simulink model "simulacao"  (R2016a)
settings: Solver=ode45  StartTime=0.0  StopTime=800  RelTol=1e-3
undefined symbols (not defined in the file or in its folder): magnitude
libraries: simulink x12
settings Model: Creator=Paulo  LastModifiedBy=Nielsen
settings DataIOCC: LimitDataPoints=on  SaveFormat=Array
settings DebuggingCC: UnderspecifiedInitializationDetection=Classic  MergeDetectMultiDrivingBlocksExec=none  SolverPrmCheckMsg=warning  StateNameClashWarn=warning
settings HardwareCC: ProdBitPerPointer=32  ProdLargestAtomicFloat=None  ProdIntDivRoundTo=Undefined  ProdEndianess=Unspecified  ProdWordSize=32  ProdHWDeviceType=32-bit Generic
settings ModelReferenceCC: PropagateSignalLabelsOutOfModel=off
settings ConfigComp: CovModelRefEnable=Off

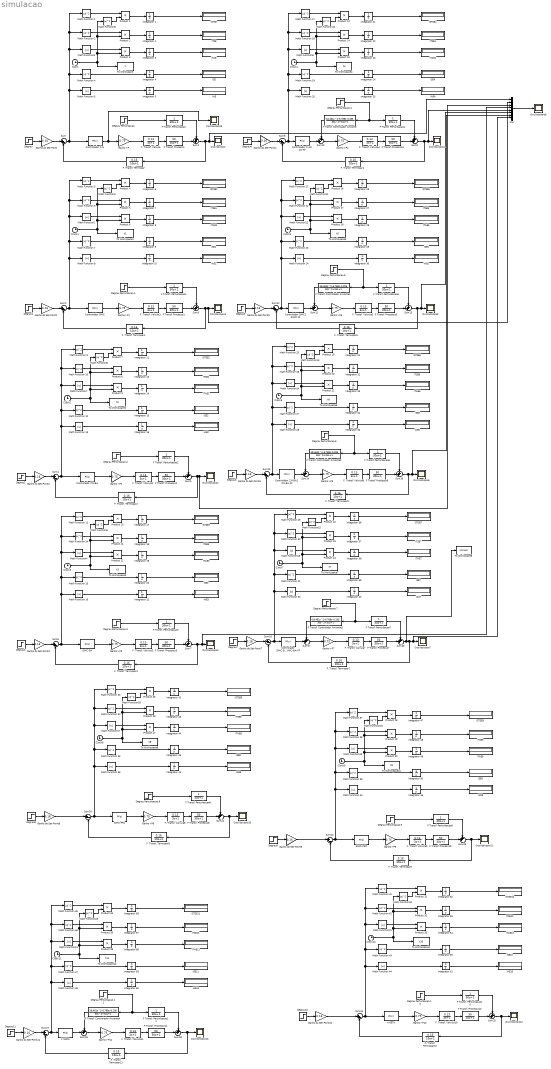
== system simulacao ==
  Clock{,1..11} (12 alike) : Clock
  Controlador SIMC : simulink/Continuous/PID Controller  Controller=PI  TimeDomain=Continuous-time  SampleTime=-1  IntegratorMethod=Forward Euler  FilterMethod=Forward Euler  Form=Parallel  UseFilter=on  ControllerParametersSource=internal  P=2.6618  I=0.0919  D=0  N=100  InitialConditionSource=internal  InitialConditionForIntegrator=0  InitialConditionForFilter=0  ExternalReset=none  LimitOutput=off  UpperSaturationLimit=10  LowerSaturationLimit=-10  LinearizeAsGain=on  AntiWindupMode=back-calculation  Kb=1  TrackingMode=off  Kt=1  PParamMin=[]  PParamMax=[]  IParamMin=[]  IParamMax=[]  DParamMin=[]  DParamMax=[]  NParamMin=[]  NParamMax=[]  KbParamMin=[]  KbParamMax=[]  KtParamMin=[]  KtParamMax=[]  POutMin=[]  POutMax=[]  IOutMin=[]  IOutMax=[]  DOutMin=[]  DOutMax=[]  NOutMin=[]  NOutMax=[]  KbOutMin=[]  KbOutMax=[]  KtOutMin=[]  KtOutMax=[]  IntegratorOutMin=[]  IntegratorOutMax=[]  FilterOutMin=[]  FilterOutMax=[]  SumOutMin=[]  SumOutMax=[]  SumI1OutMin=[]  SumI1OutMax=[]  SumI2OutMin=[]  SumI2OutMax=[]  SumI3OutMin=[]  SumI3OutMax=[]  SumDOutMin=[]  SumDOutMax=[]  SaturationOutMin=[]  SaturationOutMax=[]  IntegratorContinuousStateAttributes=''  IntegratorStateMustResolveToSignalObject=off  IntegratorRTWStateStorageClass=Auto  FilterContinuousStateAttributes=''  FilterStateMustResolveToSignalObject=off  FilterRTWStateStorageClass=Auto  DifferentiatorICPrevScaledInput=0  DifferentiatorOutMin=[]  DifferentiatorOutMax=[]
  Controlador SIMC-BA2 SIMIC-BA-FF : simulink/Continuous/PID Controller  Controller=PI  TimeDomain=Continuous-time  SampleTime=-1  IntegratorMethod=Forward Euler  FilterMethod=Forward Euler  Form=Parallel  UseFilter=on  ControllerParametersSource=internal  P=2.0483  I=0.054208  D=0  N=100  InitialConditionSource=internal  InitialConditionForIntegrator=0  InitialConditionForFilter=0  ExternalReset=none  LimitOutput=off  UpperSaturationLimit=10  LowerSaturationLimit=-10  LinearizeAsGain=on  AntiWindupMode=back-calculation  Kb=1  TrackingMode=off  Kt=1  PParamMin=[]  PParamMax=[]  IParamMin=[]  IParamMax=[]  DParamMin=[]  DParamMax=[]  NParamMin=[]  NParamMax=[]  KbParamMin=[]  KbParamMax=[]  KtParamMin=[]  KtParamMax=[]  POutMin=[]  POutMax=[]  IOutMin=[]  IOutMax=[]  DOutMin=[]  DOutMax=[]  NOutMin=[]  NOutMax=[]  KbOutMin=[]  KbOutMax=[]  KtOutMin=[]  KtOutMax=[]  IntegratorOutMin=[]  IntegratorOutMax=[]  FilterOutMin=[]  FilterOutMax=[]  SumOutMin=[]  SumOutMax=[]  SumI1OutMin=[]  SumI1OutMax=[]  SumI2OutMin=[]  SumI2OutMax=[]  SumI3OutMin=[]  SumI3OutMax=[]  SumDOutMin=[]  SumDOutMax=[]  SaturationOutMin=[]  SaturationOutMax=[]  IntegratorContinuousStateAttributes=''  IntegratorStateMustResolveToSignalObject=off  IntegratorRTWStateStorageClass=Auto  FilterContinuousStateAttributes=''  FilterStateMustResolveToSignalObject=off  FilterRTWStateStorageClass=Auto  DifferentiatorICPrevScaledInput=0  DifferentiatorOutMin=[]  DifferentiatorOutMax=[]
  "Controlador SIMC2 SIMIC FF " : simulink/Continuous/PID Controller  Controller=PI  TimeDomain=Continuous-time  SampleTime=-1  IntegratorMethod=Forward Euler  FilterMethod=Forward Euler  Form=Parallel  UseFilter=on  ControllerParametersSource=internal  P=2.6618  I=0.0919  D=0  N=100  InitialConditionSource=internal  InitialConditionForIntegrator=0  InitialConditionForFilter=0  ExternalReset=none  LimitOutput=off  UpperSaturationLimit=10  LowerSaturationLimit=-10  LinearizeAsGain=on  AntiWindupMode=back-calculation  Kb=1  TrackingMode=off  Kt=1  PParamMin=[]  PParamMax=[]  IParamMin=[]  IParamMax=[]  DParamMin=[]  DParamMax=[]  NParamMin=[]  NParamMax=[]  KbParamMin=[]  KbParamMax=[]  KtParamMin=[]  KtParamMax=[]  POutMin=[]  POutMax=[]  IOutMin=[]  IOutMax=[]  DOutMin=[]  DOutMax=[]  NOutMin=[]  NOutMax=[]  KbOutMin=[]  KbOutMax=[]  KtOutMin=[]  KtOutMax=[]  IntegratorOutMin=[]  IntegratorOutMax=[]  FilterOutMin=[]  FilterOutMax=[]  SumOutMin=[]  SumOutMax=[]  SumI1OutMin=[]  SumI1OutMax=[]  SumI2OutMin=[]  SumI2OutMax=[]  SumI3OutMin=[]  SumI3OutMax=[]  SumDOutMin=[]  SumDOutMax=[]  SaturationOutMin=[]  SaturationOutMax=[]  IntegratorContinuousStateAttributes=''  IntegratorStateMustResolveToSignalObject=off  IntegratorRTWStateStorageClass=Auto  FilterContinuousStateAttributes=''  FilterStateMustResolveToSignalObject=off  FilterRTWStateStorageClass=Auto  DifferentiatorICPrevScaledInput=0  DifferentiatorOutMin=[]  DifferentiatorOutMax=[]
  Controlador Z-N : simulink/Continuous/PID Controller  Controller=PI  TimeDomain=Continuous-time  SampleTime=-1  IntegratorMethod=Forward Euler  FilterMethod=Forward Euler  Form=Parallel  UseFilter=on  ControllerParametersSource=internal  P=10.71  I=0.437  D=0  N=100  InitialConditionSource=internal  InitialConditionForIntegrator=0  InitialConditionForFilter=0  ExternalReset=none  LimitOutput=off  UpperSaturationLimit=10  LowerSaturationLimit=-10  LinearizeAsGain=on  AntiWindupMode=back-calculation  Kb=1  TrackingMode=off  Kt=1  PParamMin=[]  PParamMax=[]  IParamMin=[]  IParamMax=[]  DParamMin=[]  DParamMax=[]  NParamMin=[]  NParamMax=[]  KbParamMin=[]  KbParamMax=[]  KtParamMin=[]  KtParamMax=[]  POutMin=[]  POutMax=[]  IOutMin=[]  IOutMax=[]  DOutMin=[]  DOutMax=[]  NOutMin=[]  NOutMax=[]  KbOutMin=[]  KbOutMax=[]  KtOutMin=[]  KtOutMax=[]  IntegratorOutMin=[]  IntegratorOutMax=[]  FilterOutMin=[]  FilterOutMax=[]  SumOutMin=[]  SumOutMax=[]  SumI1OutMin=[]  SumI1OutMax=[]  SumI2OutMin=[]  SumI2OutMax=[]  SumI3OutMin=[]  SumI3OutMax=[]  SumDOutMin=[]  SumDOutMax=[]  SaturationOutMin=[]  SaturationOutMax=[]  IntegratorContinuousStateAttributes=''  IntegratorStateMustResolveToSignalObject=off  IntegratorRTWStateStorageClass=Auto  FilterContinuousStateAttributes=''  FilterStateMustResolveToSignalObject=off  FilterRTWStateStorageClass=Auto  DifferentiatorICPrevScaledInput=0  DifferentiatorOutMin=[]  DifferentiatorOutMax=[]
  Controlador Z-N2 ZN-FF : simulink/Continuous/PID Controller  Controller=PI  TimeDomain=Continuous-time  SampleTime=-1  IntegratorMethod=Forward Euler  FilterMethod=Forward Euler  Form=Parallel  UseFilter=on  ControllerParametersSource=internal  P=10.71  I=0.437  D=0  N=100  InitialConditionSource=internal  InitialConditionForIntegrator=0  InitialConditionForFilter=0  ExternalReset=none  LimitOutput=off  UpperSaturationLimit=10  LowerSaturationLimit=-10  LinearizeAsGain=on  AntiWindupMode=back-calculation  Kb=1  TrackingMode=off  Kt=1  PParamMin=[]  PParamMax=[]  IParamMin=[]  IParamMax=[]  DParamMin=[]  DParamMax=[]  NParamMin=[]  NParamMax=[]  KbParamMin=[]  KbParamMax=[]  KtParamMin=[]  KtParamMax=[]  POutMin=[]  POutMax=[]  IOutMin=[]  IOutMax=[]  DOutMin=[]  DOutMax=[]  NOutMin=[]  NOutMax=[]  KbOutMin=[]  KbOutMax=[]  KtOutMin=[]  KtOutMax=[]  IntegratorOutMin=[]  IntegratorOutMax=[]  FilterOutMin=[]  FilterOutMax=[]  SumOutMin=[]  SumOutMax=[]  SumI1OutMin=[]  SumI1OutMax=[]  SumI2OutMin=[]  SumI2OutMax=[]  SumI3OutMin=[]  SumI3OutMax=[]  SumDOutMin=[]  SumDOutMax=[]  SaturationOutMin=[]  SaturationOutMax=[]  IntegratorContinuousStateAttributes=''  IntegratorStateMustResolveToSignalObject=off  IntegratorRTWStateStorageClass=Auto  FilterContinuousStateAttributes=''  FilterStateMustResolveToSignalObject=off  FilterRTWStateStorageClass=Auto  DifferentiatorICPrevScaledInput=0  DifferentiatorOutMin=[]  DifferentiatorOutMax=[]
  Controlador ZN-BA : simulink/Continuous/PID Controller  Controller=PI  TimeDomain=Continuous-time  SampleTime=-1  IntegratorMethod=Forward Euler  FilterMethod=Forward Euler  Form=Parallel  UseFilter=on  ControllerParametersSource=internal  P=5.355  I=0.2185  D=0  N=100  InitialConditionSource=internal  InitialConditionForIntegrator=0  InitialConditionForFilter=0  ExternalReset=none  LimitOutput=off  UpperSaturationLimit=10  LowerSaturationLimit=-10  LinearizeAsGain=on  AntiWindupMode=back-calculation  Kb=1  TrackingMode=off  Kt=1  PParamMin=[]  PParamMax=[]  IParamMin=[]  IParamMax=[]  DParamMin=[]  DParamMax=[]  NParamMin=[]  NParamMax=[]  KbParamMin=[]  KbParamMax=[]  KtParamMin=[]  KtParamMax=[]  POutMin=[]  POutMax=[]  IOutMin=[]  IOutMax=[]  DOutMin=[]  DOutMax=[]  NOutMin=[]  NOutMax=[]  KbOutMin=[]  KbOutMax=[]  KtOutMin=[]  KtOutMax=[]  IntegratorOutMin=[]  IntegratorOutMax=[]  FilterOutMin=[]  FilterOutMax=[]  SumOutMin=[]  SumOutMax=[]  SumI1OutMin=[]  SumI1OutMax=[]  SumI2OutMin=[]  SumI2OutMax=[]  SumI3OutMin=[]  SumI3OutMax=[]  SumDOutMin=[]  SumDOutMax=[]  SaturationOutMin=[]  SaturationOutMax=[]  IntegratorContinuousStateAttributes=''  IntegratorStateMustResolveToSignalObject=off  IntegratorRTWStateStorageClass=Auto  FilterContinuousStateAttributes=''  FilterStateMustResolveToSignalObject=off  FilterRTWStateStorageClass=Auto  DifferentiatorICPrevScaledInput=0  DifferentiatorOutMin=[]  DifferentiatorOutMax=[]
  Controlador ZN-BA2 ZN-BA-FF : simulink/Continuous/PID Controller  Controller=PI  TimeDomain=Continuous-time  SampleTime=-1  IntegratorMethod=Forward Euler  FilterMethod=Forward Euler  Form=Parallel  UseFilter=on  ControllerParametersSource=internal  P=5.355  I=0.2185  D=0  N=100  InitialConditionSource=internal  InitialConditionForIntegrator=0  InitialConditionForFilter=0  ExternalReset=none  LimitOutput=off  UpperSaturationLimit=10  LowerSaturationLimit=-10  LinearizeAsGain=on  AntiWindupMode=back-calculation  Kb=1  TrackingMode=off  Kt=1  PParamMin=[]  PParamMax=[]  IParamMin=[]  IParamMax=[]  DParamMin=[]  DParamMax=[]  NParamMin=[]  NParamMax=[]  KbParamMin=[]  KbParamMax=[]  KtParamMin=[]  KtParamMax=[]  POutMin=[]  POutMax=[]  IOutMin=[]  IOutMax=[]  DOutMin=[]  DOutMax=[]  NOutMin=[]  NOutMax=[]  KbOutMin=[]  KbOutMax=[]  KtOutMin=[]  KtOutMax=[]  IntegratorOutMin=[]  IntegratorOutMax=[]  FilterOutMin=[]  FilterOutMax=[]  SumOutMin=[]  SumOutMax=[]  SumI1OutMin=[]  SumI1OutMax=[]  SumI2OutMin=[]  SumI2OutMax=[]  SumI3OutMin=[]  SumI3OutMax=[]  SumDOutMin=[]  SumDOutMax=[]  SaturationOutMin=[]  SaturationOutMax=[]  IntegratorContinuousStateAttributes=''  IntegratorStateMustResolveToSignalObject=off  IntegratorRTWStateStorageClass=Auto  FilterContinuousStateAttributes=''  FilterStateMustResolveToSignalObject=off  FilterRTWStateStorageClass=Auto  DifferentiatorICPrevScaledInput=0  DifferentiatorOutMin=[]  DifferentiatorOutMax=[]
  Degrau{,1..11} (12 alike) : Step  Time=0  SampleTime=0
  Degrau Perturbacao.{,1..11} (12 alike) : Step  Time=0  SampleTime=0
  F Transf. Controlador Anvante{,1..4} (5 alike) : TransferFcn  Numerator=[-18.461 -6.769 -0.205]  Denominator=[30 31 1]
  F Transf. Perturbacao{,1..11} (12 alike) : TransferFcn  Denominator=[30 1]
  F Transf. Processo{,1..11} (12 alike) : TransferFcn  Numerator=[50]  Denominator=[30 1]
  F. Transf. Termopar{,1..11} (12 alike) : TransferFcn  Numerator=[0.16]  Denominator=[10 1]
  F. Transf. Válvula{,1..11} (12 alike) : TransferFcn  Numerator=[0.13]  Denominator=[3 1]
  Ganho I-P{,1..11} (12 alike) : Gain  Gain=0.75
  Ganho do Set-Point{,1..11} (12 alike) : Gain  Gain=0.16
  IAE{,1..11} (12 alike) : Display
  ISE{,1..11} (12 alike) : Display
  ISTSE{,1..11} (12 alike) : Display
  ITAE{,1..11} (12 alike) : Display
  ITSE{,1..11} (12 alike) : Display
  Integrator {1..60} (60 alike) : Integrator
  Math Function {1..4,6..7,9..12,14..15,17..19,21..23,25..27,29..31,33..35,37..39,41..43,45..47} (36 alike) : Math  Operator=magnitude^2  SaturateOnIntegerOverflow=on
  Math Function {5,8,13,16,20,24,28,32,36,40,44,48} (12 alike) : Abs
  Math Function{1,3..4,7,9,12,14,16..17,19,21,24} (12 alike) : Abs
  Math Function{2,5..6,8,10..11,13,15,18,20,22..23} (12 alike) : Math  Operator=magnitude^2  SaturateOnIntegerOverflow=on
  Mux : Mux  Inputs=8
  Osciloscópio{,1..13} (14 alike) : Scope
  Product {1..36} (36 alike) : Product
  SIMC-BA : simulink/Continuous/PID Controller  Controller=PI  TimeDomain=Continuous-time  SampleTime=-1  IntegratorMethod=Forward Euler  FilterMethod=Forward Euler  Form=Parallel  UseFilter=on  ControllerParametersSource=internal  P=2.0483  I=0.054208  D=0  N=100  InitialConditionSource=internal  InitialConditionForIntegrator=0  InitialConditionForFilter=0  ExternalReset=none  LimitOutput=off  UpperSaturationLimit=10  LowerSaturationLimit=-10  LinearizeAsGain=on  AntiWindupMode=back-calculation  Kb=1  TrackingMode=off  Kt=1  PParamMin=[]  PParamMax=[]  IParamMin=[]  IParamMax=[]  DParamMin=[]  DParamMax=[]  NParamMin=[]  NParamMax=[]  KbParamMin=[]  KbParamMax=[]  KtParamMin=[]  KtParamMax=[]  POutMin=[]  POutMax=[]  IOutMin=[]  IOutMax=[]  DOutMin=[]  DOutMax=[]  NOutMin=[]  NOutMax=[]  KbOutMin=[]  KbOutMax=[]  KtOutMin=[]  KtOutMax=[]  IntegratorOutMin=[]  IntegratorOutMax=[]  FilterOutMin=[]  FilterOutMax=[]  SumOutMin=[]  SumOutMax=[]  SumI1OutMin=[]  SumI1OutMax=[]  SumI2OutMin=[]  SumI2OutMax=[]  SumI3OutMin=[]  SumI3OutMax=[]  SumDOutMin=[]  SumDOutMax=[]  SaturationOutMin=[]  SaturationOutMax=[]  IntegratorContinuousStateAttributes=''  IntegratorStateMustResolveToSignalObject=off  IntegratorRTWStateStorageClass=Auto  FilterContinuousStateAttributes=''  FilterStateMustResolveToSignalObject=off  FilterRTWStateStorageClass=Auto  DifferentiatorICPrevScaledInput=0  DifferentiatorOutMin=[]  DifferentiatorOutMax=[]
  SIMC-FPA : simulink/Continuous/PID Controller  Controller=PI  TimeDomain=Continuous-time  SampleTime=-1  IntegratorMethod=Forward Euler  FilterMethod=Forward Euler  Form=Parallel  UseFilter=on  ControllerParametersSource=internal  P=5.7554  I=0.2185  D=0  N=100  InitialConditionSource=internal  InitialConditionForIntegrator=0  InitialConditionForFilter=0  ExternalReset=none  LimitOutput=off  UpperSaturationLimit=10  LowerSaturationLimit=-10  LinearizeAsGain=on  AntiWindupMode=back-calculation  Kb=1  TrackingMode=off  Kt=1  PParamMin=[]  PParamMax=[]  IParamMin=[]  IParamMax=[]  DParamMin=[]  DParamMax=[]  NParamMin=[]  NParamMax=[]  KbParamMin=[]  KbParamMax=[]  KtParamMin=[]  KtParamMax=[]  POutMin=[]  POutMax=[]  IOutMin=[]  IOutMax=[]  DOutMin=[]  DOutMax=[]  NOutMin=[]  NOutMax=[]  KbOutMin=[]  KbOutMax=[]  KtOutMin=[]  KtOutMax=[]  IntegratorOutMin=[]  IntegratorOutMax=[]  FilterOutMin=[]  FilterOutMax=[]  SumOutMin=[]  SumOutMax=[]  SumI1OutMin=[]  SumI1OutMax=[]  SumI2OutMin=[]  SumI2OutMax=[]  SumI3OutMin=[]  SumI3OutMax=[]  SumDOutMin=[]  SumDOutMax=[]  SaturationOutMin=[]  SaturationOutMax=[]  IntegratorContinuousStateAttributes=''  IntegratorStateMustResolveToSignalObject=off  IntegratorRTWStateStorageClass=Auto  FilterContinuousStateAttributes=''  FilterStateMustResolveToSignalObject=off  FilterRTWStateStorageClass=Auto  DifferentiatorICPrevScaledInput=0  DifferentiatorOutMin=[]  DifferentiatorOutMax=[]
  SIMC-PSO : simulink/Continuous/PID Controller  Controller=PI  TimeDomain=Continuous-time  SampleTime=-1  IntegratorMethod=Forward Euler  FilterMethod=Forward Euler  Form=Parallel  UseFilter=on  ControllerParametersSource=internal  P=1.8638  I=0.0505  D=0  N=100  InitialConditionSource=internal  InitialConditionForIntegrator=0  InitialConditionForFilter=0  ExternalReset=none  LimitOutput=off  UpperSaturationLimit=10  LowerSaturationLimit=-10  LinearizeAsGain=on  AntiWindupMode=back-calculation  Kb=1  TrackingMode=off  Kt=1  PParamMin=[]  PParamMax=[]  IParamMin=[]  IParamMax=[]  DParamMin=[]  DParamMax=[]  NParamMin=[]  NParamMax=[]  KbParamMin=[]  KbParamMax=[]  KtParamMin=[]  KtParamMax=[]  POutMin=[]  POutMax=[]  IOutMin=[]  IOutMax=[]  DOutMin=[]  DOutMax=[]  NOutMin=[]  NOutMax=[]  KbOutMin=[]  KbOutMax=[]  KtOutMin=[]  KtOutMax=[]  IntegratorOutMin=[]  IntegratorOutMax=[]  FilterOutMin=[]  FilterOutMax=[]  SumOutMin=[]  SumOutMax=[]  SumI1OutMin=[]  SumI1OutMax=[]  SumI2OutMin=[]  SumI2OutMax=[]  SumI3OutMin=[]  SumI3OutMax=[]  SumDOutMin=[]  SumDOutMax=[]  SaturationOutMin=[]  SaturationOutMax=[]  IntegratorContinuousStateAttributes=''  IntegratorStateMustResolveToSignalObject=off  IntegratorRTWStateStorageClass=Auto  FilterContinuousStateAttributes=''  FilterStateMustResolveToSignalObject=off  FilterRTWStateStorageClass=Auto  DifferentiatorICPrevScaledInput=0  DifferentiatorOutMin=[]  DifferentiatorOutMax=[]
  Sum{,2,4,6,8,12,15,18,20,22,24,27} (12 alike) : Sum  Inputs=|+-
  Sum{1,3,5,7,9..11,13..14,16..17,19,21,23,25..26,28} (17 alike) : Sum  Inputs=++|
  To Workspace : ToWorkspace  VariableName=t  SampleTime=-1
  To Workspace1 : ToWorkspace  VariableName=t1  SampleTime=-1
  To Workspace10 : ToWorkspace  VariableName=t9  SampleTime=-1
  To Workspace11 : ToWorkspace  VariableName=t10  SampleTime=-1
  To Workspace12 : ToWorkspace  VariableName=t11  SampleTime=-1
  To Workspace2 : ToWorkspace  VariableName=t2  SampleTime=-1
  To Workspace3 : ToWorkspace  VariableName=t3  SampleTime=-1
  To Workspace4 : ToWorkspace  VariableName=t4  SampleTime=-1
  To Workspace5 : ToWorkspace  VariableName=t5  SampleTime=-1
  To Workspace6 : ToWorkspace  VariableName=t6  SampleTime=-1
  To Workspace7 : ToWorkspace  VariableName=t7  SampleTime=-1
  To Workspace8 : ToWorkspace  VariableName=simout  SampleTime=-1
  To Workspace9 : ToWorkspace  VariableName=t8  SampleTime=-1
  X META : simulink/Continuous/PID Controller  Controller=PI  TimeDomain=Continuous-time  SampleTime=-1  IntegratorMethod=Forward Euler  FilterMethod=Forward Euler  Form=Parallel  UseFilter=on  ControllerParametersSource=internal  P=10.71  I=0.437  D=0  N=100  InitialConditionSource=internal  InitialConditionForIntegrator=0  InitialConditionForFilter=0  ExternalReset=none  LimitOutput=off  UpperSaturationLimit=10  LowerSaturationLimit=-10  LinearizeAsGain=on  AntiWindupMode=back-calculation  Kb=1  TrackingMode=off  Kt=1  PParamMin=[]  PParamMax=[]  IParamMin=[]  IParamMax=[]  DParamMin=[]  DParamMax=[]  NParamMin=[]  NParamMax=[]  KbParamMin=[]  KbParamMax=[]  KtParamMin=[]  KtParamMax=[]  POutMin=[]  POutMax=[]  IOutMin=[]  IOutMax=[]  DOutMin=[]  DOutMax=[]  NOutMin=[]  NOutMax=[]  KbOutMin=[]  KbOutMax=[]  KtOutMin=[]  KtOutMax=[]  IntegratorOutMin=[]  IntegratorOutMax=[]  FilterOutMin=[]  FilterOutMax=[]  SumOutMin=[]  SumOutMax=[]  SumI1OutMin=[]  SumI1OutMax=[]  SumI2OutMin=[]  SumI2OutMax=[]  SumI3OutMin=[]  SumI3OutMax=[]  SumDOutMin=[]  SumDOutMax=[]  SaturationOutMin=[]  SaturationOutMax=[]  IntegratorContinuousStateAttributes=''  IntegratorStateMustResolveToSignalObject=off  IntegratorRTWStateStorageClass=Auto  FilterContinuousStateAttributes=''  FilterStateMustResolveToSignalObject=off  FilterRTWStateStorageClass=Auto  DifferentiatorICPrevScaledInput=0  DifferentiatorOutMin=[]  DifferentiatorOutMax=[]
  XMETA : simulink/Continuous/PID Controller  Controller=PI  TimeDomain=Continuous-time  SampleTime=-1  IntegratorMethod=Forward Euler  FilterMethod=Forward Euler  Form=Parallel  UseFilter=on  ControllerParametersSource=internal  P=5.2114  I=0.1140  D=0  N=100  InitialConditionSource=internal  InitialConditionForIntegrator=0  InitialConditionForFilter=0  ExternalReset=none  LimitOutput=off  UpperSaturationLimit=10  LowerSaturationLimit=-10  LinearizeAsGain=on  AntiWindupMode=back-calculation  Kb=1  TrackingMode=off  Kt=1  PParamMin=[]  PParamMax=[]  IParamMin=[]  IParamMax=[]  DParamMin=[]  DParamMax=[]  NParamMin=[]  NParamMax=[]  KbParamMin=[]  KbParamMax=[]  KtParamMin=[]  KtParamMax=[]  POutMin=[]  POutMax=[]  IOutMin=[]  IOutMax=[]  DOutMin=[]  DOutMax=[]  NOutMin=[]  NOutMax=[]  KbOutMin=[]  KbOutMax=[]  KtOutMin=[]  KtOutMax=[]  IntegratorOutMin=[]  IntegratorOutMax=[]  FilterOutMin=[]  FilterOutMax=[]  SumOutMin=[]  SumOutMax=[]  SumI1OutMin=[]  SumI1OutMax=[]  SumI2OutMin=[]  SumI2OutMax=[]  SumI3OutMin=[]  SumI3OutMax=[]  SumDOutMin=[]  SumDOutMax=[]  SaturationOutMin=[]  SaturationOutMax=[]  IntegratorContinuousStateAttributes=''  IntegratorStateMustResolveToSignalObject=off  IntegratorRTWStateStorageClass=Auto  FilterContinuousStateAttributes=''  FilterStateMustResolveToSignalObject=off  FilterRTWStateStorageClass=Auto  DifferentiatorICPrevScaledInput=0  DifferentiatorOutMin=[]  DifferentiatorOutMax=[]
  wires:
  Degrau/1 -> Ganho do Set-Point/1
  Ganho do Set-Point/1 -> Sum/1
  Ganho I-P/1 -> F. Transf. Válvula/1
  F. Transf. Válvula/1 -> F Transf. Processo/1
  F. Transf. Termopar/1 -> Sum/2
  F Transf. Perturbacao/1 -> Sum1/1
  F Transf. Processo/1 -> Sum1/2
  Degrau Perturbacao./1 -> F Transf. Perturbacao/1
  Sum/1 -> Math Function 5/1, Math Function 4/1, Math Function3/1, Math Function 2/1, Math Function 1/1, Controlador Z-N/1
  Product 1/1 -> Integrator 1/1
  Product 2/1 -> Integrator 2/1
  Product 3/1 -> Integrator 3/1
  Math Function3/1 -> Product 3/1
  Math Function 1/1 -> Product 1/1
  Math Function 2/1 -> Product 2/1
  Integrator 1/1 -> ISTSE/1
  Integrator 2/1 -> ITSE/1
  Integrator 3/1 -> ITAE/1
  Math Function 4/1 -> Integrator 4/1
  Math Function 5/1 -> Integrator 5/1
  Clock/1 -> Product 3/2, Product 2/2, Math Function6/1, To Workspace/1
  Math Function6/1 -> Product 1/2
  Integrator 4/1 -> ISE/1
  Integrator 5/1 -> IAE/1
  Degrau1/1 -> Ganho do Set-Point1/1
  Ganho do Set-Point1/1 -> Sum2/1
  Ganho I-P1/1 -> F. Transf. Válvula1/1
  F. Transf. Válvula1/1 -> F Transf. Processo1/1
  F. Transf. Termopar1/1 -> Sum2/2
  F Transf. Perturbacao1/1 -> Sum3/1
  F Transf. Processo1/1 -> Sum3/2
  Degrau Perturbacao.1/1 -> F Transf. Perturbacao1/1
  Sum2/1 -> Math Function 8/1, Math Function 7/1, Math Function1/1, Math Function 6/1, Math Function 3/1, Controlador SIMC/1
  Product 4/1 -> Integrator 6/1
  Product 5/1 -> Integrator 7/1
  Product 6/1 -> Integrator 8/1
  Math Function1/1 -> Product 6/1
  Math Function 3/1 -> Product 4/1
  Math Function 6/1 -> Product 5/1
  Integrator 6/1 -> ISTSE1/1
  Integrator 7/1 -> ITSE1/1
  Integrator 8/1 -> ITAE1/1
  Math Function 7/1 -> Integrator 9/1
  Math Function 8/1 -> Integrator 10/1
  Clock1/1 -> Product 6/2, Product 5/2, Math Function2/1, To Workspace1/1
  Math Function2/1 -> Product 4/2
  Integrator 9/1 -> ISE1/1
  Integrator 10/1 -> IAE1/1
  Controlador SIMC/1 -> Ganho I-P1/1
  Degrau2/1 -> Ganho do Set-Point2/1
  Ganho do Set-Point2/1 -> Sum4/1
  Ganho I-P2/1 -> F. Transf. Válvula2/1
  F. Transf. Válvula2/1 -> F Transf. Processo2/1
  F. Transf. Termopar2/1 -> Sum4/2
  F Transf. Perturbacao2/1 -> Sum5/1
  F Transf. Processo2/1 -> Sum5/2
  Degrau Perturbacao.2/1 -> F Transf. Perturbacao2/1
  Sum4/1 -> Math Function 13/1, Math Function 12/1, Math Function7/1, Math Function 10/1, Math Function 9/1, Controlador ZN-BA/1
  Product 7/1 -> Integrator 11/1
  Product 8/1 -> Integrator 13/1
  Product 9/1 -> Integrator 14/1
  Math Function7/1 -> Product 9/1
  Math Function 9/1 -> Product 7/1
  Math Function 10/1 -> Product 8/1
  Integrator 11/1 -> ISTSE2/1
  Integrator 13/1 -> ITSE2/1
  Integrator 14/1 -> ITAE2/1
  Math Function 12/1 -> Integrator 15/1
  Math Function 13/1 -> Integrator 16/1
  Clock2/1 -> Product 9/2, Product 8/2, Math Function8/1, To Workspace2/1
  Math Function8/1 -> Product 7/2
  Integrator 15/1 -> ISE2/1
  Integrator 16/1 -> IAE2/1
  Controlador ZN-BA/1 -> Ganho I-P2/1
  Degrau3/1 -> Ganho do Set-Point3/1
  Ganho do Set-Point3/1 -> Sum6/1
  Ganho I-P3/1 -> F. Transf. Válvula3/1
  F. Transf. Válvula3/1 -> F Transf. Processo3/1
  F. Transf. Termopar3/1 -> Sum6/2
  F Transf. Processo3/1 -> Sum7/2
  Degrau Perturbacao.3/1 -> F Transf. Perturbacao3/1
  Sum6/1 -> Math Function 16/1, Math Function 15/1, Math Function4/1, Math Function 14/1, Math Function 11/1, SIMC-BA/1
  Product 10/1 -> Integrator 17/1
  Product 11/1 -> Integrator 18/1
  Product 12/1 -> Integrator 19/1
  Math Function4/1 -> Product 12/1
  Math Function 11/1 -> Product 10/1
  Math Function 14/1 -> Product 11/1
  Integrator 17/1 -> ISTSE3/1
  Integrator 18/1 -> ITSE3/1
  Integrator 19/1 -> ITAE3/1
  Math Function 15/1 -> Integrator 20/1
  Math Function 16/1 -> Integrator 12/1
  Clock3/1 -> Product 12/2, Product 11/2, Math Function5/1, To Workspace3/1
  Math Function5/1 -> Product 10/2
  Integrator 20/1 -> ISE3/1
  Integrator 12/1 -> IAE3/1
  SIMC-BA/1 -> Ganho I-P3/1
  Degrau4/1 -> Ganho do Set-Point4/1
  Ganho do Set-Point4/1 -> Sum8/1
  Ganho I-P4/1 -> F. Transf. Válvula4/1
  F. Transf. Válvula4/1 -> F Transf. Processo4/1
  F. Transf. Termopar4/1 -> Sum8/2
  F Transf. Perturbacao4/1 -> Sum9/1
  Sum10/1 -> Ganho I-P4/1
  Controlador Z-N2 ZN-FF/1 -> Sum10/2
  F Transf. Controlador Anvante/1 -> Sum10/1
  F Transf. Processo4/1 -> Sum9/2
  Degrau Perturbacao.4/1 -> F Transf. Controlador Anvante/1, F Transf. Perturbacao4/1
  Sum8/1 -> Math Function 20/1, Math Function 19/1, Math Function9/1, Math Function 18/1, Math Function 17/1, Controlador Z-N2 ZN-FF/1
  Product 13/1 -> Integrator 21/1
  Product 14/1 -> Integrator 22/1
  Product 15/1 -> Integrator 23/1
  Math Function9/1 -> Product 15/1
  Math Function 17/1 -> Product 13/1
  Math Function 18/1 -> Product 14/1
  Integrator 21/1 -> ISTSE4/1
  Integrator 22/1 -> ITSE4/1
  Integrator 23/1 -> ITAE4/1
  Math Function 19/1 -> Integrator 24/1
  Math Function 20/1 -> Integrator 25/1
  Clock4/1 -> Product 15/2, Product 14/2, Math Function10/1, To Workspace4/1
  Math Function10/1 -> Product 13/2
  Integrator 24/1 -> ISE4/1
  Integrator 25/1 -> IAE4/1
  Degrau5/1 -> Ganho do Set-Point5/1
  Ganho do Set-Point5/1 -> Sum12/1
  Ganho I-P5/1 -> F. Transf. Válvula5/1
  F. Transf. Válvula5/1 -> F Transf. Processo5/1
  F. Transf. Termopar5/1 -> Sum12/2
  F Transf. Perturbacao5/1 -> Sum13/1
  Sum11/1 -> Ganho I-P5/1
  "Controlador SIMC2 SIMIC FF "/1 -> Sum11/2
  F Transf. Controlador Anvante1/1 -> Sum11/1
  F Transf. Processo5/1 -> Sum13/2
  Degrau Perturbacao.5/1 -> F Transf. Controlador Anvante1/1, F Transf. Perturbacao5/1
  Sum12/1 -> Math Function 24/1, Math Function 23/1, Math Function12/1, Math Function 22/1, Math Function 21/1, "Controlador SIMC2 SIMIC FF "/1
  Product 16/1 -> Integrator 26/1
  Product 17/1 -> Integrator 27/1
  Product 18/1 -> Integrator 28/1
  Math Function12/1 -> Product 18/1
  Math Function 21/1 -> Product 16/1
  Math Function 22/1 -> Product 17/1
  Integrator 26/1 -> ISTSE5/1
  Integrator 27/1 -> ITSE5/1
  Integrator 28/1 -> ITAE5/1
  Math Function 23/1 -> Integrator 29/1
  Math Function 24/1 -> Integrator 30/1
  Clock5/1 -> Product 18/2, Product 17/2, Math Function11/1, To Workspace5/1
  Math Function11/1 -> Product 16/2
  Integrator 29/1 -> ISE5/1
  Integrator 30/1 -> IAE5/1
  Degrau6/1 -> Ganho do Set-Point6/1
  Ganho do Set-Point6/1 -> Sum15/1
  Ganho I-P6/1 -> F. Transf. Válvula6/1
  F. Transf. Válvula6/1 -> F Transf. Processo6/1
  F. Transf. Termopar6/1 -> Sum15/2
  F Transf. Perturbacao6/1 -> Sum16/1
  Sum14/1 -> Ganho I-P6/1
  Controlador ZN-BA2 ZN-BA-FF/1 -> Sum14/2
  F Transf. Controlador Anvante2/1 -> Sum14/1
  F Transf. Processo6/1 -> Sum16/2
  Degrau Perturbacao.6/1 -> F Transf. Controlador Anvante2/1, F Transf. Perturbacao6/1
  Sum15/1 -> Math Function 28/1, Math Function 27/1, Math Function14/1, Math Function 26/1, Math Function 25/1, Controlador ZN-BA2 ZN-BA-FF/1
  Product 19/1 -> Integrator 31/1
  Product 20/1 -> Integrator 32/1
  Product 21/1 -> Integrator 33/1
  Math Function14/1 -> Product 21/1
  Math Function 25/1 -> Product 19/1
  Math Function 26/1 -> Product 20/1
  Integrator 31/1 -> ISTSE6/1
  Integrator 32/1 -> ITSE6/1
  Integrator 33/1 -> ITAE6/1
  Math Function 27/1 -> Integrator 34/1
  Math Function 28/1 -> Integrator 35/1
  Clock6/1 -> Product 21/2, Product 20/2, Math Function13/1, To Workspace6/1
  Math Function13/1 -> Product 19/2
  Integrator 34/1 -> ISE6/1
  Integrator 35/1 -> IAE6/1
  Degrau7/1 -> Ganho do Set-Point7/1
  Ganho do Set-Point7/1 -> Sum18/1
  Ganho I-P7/1 -> F. Transf. Válvula7/1
  F. Transf. Válvula7/1 -> F Transf. Processo7/1
  F. Transf. Termopar7/1 -> Sum18/2
  F Transf. Perturbacao7/1 -> Sum19/1
  Sum17/1 -> Ganho I-P7/1
  Controlador SIMC-BA2 SIMIC-BA-FF/1 -> Sum17/2
  F Transf. Controlador Anvante3/1 -> Sum17/1
  F Transf. Processo7/1 -> Sum19/2
  Degrau Perturbacao.7/1 -> F Transf. Controlador Anvante3/1, F Transf. Perturbacao7/1
  Sum18/1 -> Math Function 32/1, Math Function 31/1, Math Function16/1, Math Function 30/1, Math Function 29/1, Controlador SIMC-BA2 SIMIC-BA-FF/1
  Product 22/1 -> Integrator 36/1
  Product 23/1 -> Integrator 37/1
  Product 24/1 -> Integrator 38/1
  Math Function16/1 -> Product 24/1
  Math Function 29/1 -> Product 22/1
  Math Function 30/1 -> Product 23/1
  Integrator 36/1 -> ISTSE7/1
  Integrator 37/1 -> ITSE7/1
  Integrator 38/1 -> ITAE7/1
  Math Function 31/1 -> Integrator 39/1
  Math Function 32/1 -> Integrator 40/1
  Clock7/1 -> Product 24/2, Product 23/2, Math Function15/1, To Workspace7/1
  Math Function15/1 -> Product 22/2
  Integrator 39/1 -> ISE7/1
  Integrator 40/1 -> IAE7/1
  Sum1/1 -> F. Transf. Termopar/1, Mux/1, Osciloscópio/1
  Sum3/1 -> F. Transf. Termopar1/1, Mux/2, Osciloscópio1/1
  Sum7/1 -> F. Transf. Termopar3/1, Mux/4, Osciloscópio3/1
  Sum9/1 -> F. Transf. Termopar4/1, Mux/5, Osciloscópio4/1
  Sum13/1 -> F. Transf. Termopar5/1, Mux/6, Osciloscópio5/1
  Sum16/1 -> F. Transf. Termopar6/1, Mux/7, Osciloscópio6/1
  Sum19/1 -> To Workspace8/1, F. Transf. Termopar7/1, Mux/8, Osciloscópio7/1
  Mux/1 -> Osciloscópio8/1
  Sum5/1 -> F. Transf. Termopar2/1, Mux/3, Osciloscópio2/1
  Controlador Z-N/1 -> Osciloscópio9/1, Ganho I-P/1
  F Transf. Perturbacao3/1 -> Sum7/1
  Degrau8/1 -> Ganho do Set-Point8/1
  Ganho I-P8/1 -> F. Transf. Válvula8/1
  F. Transf. Válvula8/1 -> F Transf. Processo8/1
  F. Transf. Termopar8/1 -> Sum20/2
  F Transf. Processo8/1 -> Sum21/2
  Degrau Perturbacao.8/1 -> F Transf. Perturbacao8/1
  Sum20/1 -> Math Function 36/1, Math Function 35/1, Math Function17/1, Math Function 34/1, Math Function 33/1, SIMC-FPA/1
  Product 25/1 -> Integrator 42/1
  Product 26/1 -> Integrator 43/1
  Product 27/1 -> Integrator 44/1
  Math Function17/1 -> Product 27/1
  Math Function 33/1 -> Product 25/1
  Math Function 34/1 -> Product 26/1
  Integrator 42/1 -> ISTSE8/1
  Integrator 43/1 -> ITSE8/1
  Integrator 44/1 -> ITAE8/1
  Math Function 35/1 -> Integrator 45/1
  Math Function 36/1 -> Integrator 41/1
  Clock8/1 -> Product 27/2, Product 26/2, Math Function18/1, To Workspace9/1
  Math Function18/1 -> Product 25/2
  Integrator 45/1 -> ISE8/1
  Integrator 41/1 -> IAE8/1
  SIMC-FPA/1 -> Ganho I-P8/1
  Sum21/1 -> F. Transf. Termopar8/1, Osciloscópio10/1
  F Transf. Perturbacao8/1 -> Sum21/1
  Ganho do Set-Point8/1 -> Sum20/1
  Degrau9/1 -> Ganho do Set-Point9/1
  Ganho I-P9/1 -> F. Transf. Válvula9/1
  F. Transf. Válvula9/1 -> F Transf. Processo9/1
  F. Transf. Termopar9/1 -> Sum22/2
  F Transf. Processo9/1 -> Sum23/2
  Degrau Perturbacao.9/1 -> F Transf. Perturbacao9/1
  Sum22/1 -> Math Function 40/1, Math Function 39/1, Math Function19/1, Math Function 38/1, Math Function 37/1, SIMC-PSO/1
  Product 28/1 -> Integrator 47/1
  Product 29/1 -> Integrator 48/1
  Product 30/1 -> Integrator 49/1
  Math Function19/1 -> Product 30/1
  Math Function 37/1 -> Product 28/1
  Math Function 38/1 -> Product 29/1
  Integrator 47/1 -> ISTSE9/1
  Integrator 48/1 -> ITSE9/1
  Integrator 49/1 -> ITAE9/1
  Math Function 39/1 -> Integrator 50/1
  Math Function 40/1 -> Integrator 46/1
  Clock9/1 -> Product 30/2, Product 29/2, Math Function20/1, To Workspace10/1
  Math Function20/1 -> Product 28/2
  Integrator 50/1 -> ISE9/1
  Integrator 46/1 -> IAE9/1
  SIMC-PSO/1 -> Ganho I-P9/1
  Sum23/1 -> F. Transf. Termopar9/1, Osciloscópio11/1
  F Transf. Perturbacao9/1 -> Sum23/1
  Ganho do Set-Point9/1 -> Sum22/1
  Degrau10/1 -> Ganho do Set-Point10/1
  Ganho I-P10/1 -> F. Transf. Válvula10/1
  F. Transf. Válvula10/1 -> F Transf. Processo10/1
  F. Transf. Termopar10/1 -> Sum24/2
  F Transf. Processo10/1 -> Sum25/2
  Degrau Perturbacao.10/1 -> F Transf. Perturbacao10/1
  Sum24/1 -> Math Function 44/1, Math Function 43/1, Math Function21/1, Math Function 42/1, Math Function 41/1, XMETA/1
  Product 31/1 -> Integrator 52/1
  Product 32/1 -> Integrator 53/1
  Product 33/1 -> Integrator 54/1
  Math Function21/1 -> Product 33/1
  Math Function 41/1 -> Product 31/1
  Math Function 42/1 -> Product 32/1
  Integrator 52/1 -> ISTSE10/1
  Integrator 53/1 -> ITSE10/1
  Integrator 54/1 -> ITAE10/1
  Math Function 43/1 -> Integrator 55/1
  Math Function 44/1 -> Integrator 51/1
  Clock10/1 -> Product 33/2, Product 32/2, Math Function22/1, To Workspace11/1
  Math Function22/1 -> Product 31/2
  Integrator 55/1 -> ISE10/1
  Integrator 51/1 -> IAE10/1
  XMETA/1 -> Ganho I-P10/1
  Sum25/1 -> F. Transf. Termopar10/1, Osciloscópio12/1
  F Transf. Perturbacao10/1 -> Sum25/1
  Ganho do Set-Point10/1 -> Sum24/1
  Degrau11/1 -> Ganho do Set-Point11/1
  Ganho do Set-Point11/1 -> Sum27/1
  Ganho I-P11/1 -> F. Transf. Válvula11/1
  F. Transf. Válvula11/1 -> F Transf. Processo11/1
  F. Transf. Termopar11/1 -> Sum27/2
  F Transf. Perturbacao11/1 -> Sum28/1
  Sum26/1 -> Ganho I-P11/1
  X META/1 -> Sum26/2
  F Transf. Controlador Anvante4/1 -> Sum26/1
  F Transf. Processo11/1 -> Sum28/2
  Degrau Perturbacao.11/1 -> F Transf. Controlador Anvante4/1, F Transf. Perturbacao11/1
  Sum27/1 -> Math Function 48/1, Math Function 47/1, Math Function24/1, Math Function 46/1, Math Function 45/1, X META/1
  Product 34/1 -> Integrator 56/1
  Product 35/1 -> Integrator 57/1
  Product 36/1 -> Integrator 58/1
  Math Function24/1 -> Product 36/1
  Math Function 45/1 -> Product 34/1
  Math Function 46/1 -> Product 35/1
  Integrator 56/1 -> ISTSE11/1
  Integrator 57/1 -> ITSE11/1
  Integrator 58/1 -> ITAE11/1
  Math Function 47/1 -> Integrator 59/1
  Math Function 48/1 -> Integrator 60/1
  Clock11/1 -> Product 36/2, Product 35/2, Math Function23/1, To Workspace12/1
  Math Function23/1 -> Product 34/2
  Integrator 59/1 -> ISE11/1
  Integrator 60/1 -> IAE11/1
  Sum28/1 -> F. Transf. Termopar11/1, Osciloscópio13/1
